simulink model "lab5_2_simulink"  (R2018a)
settings: Solver=VariableStepAuto  StartTime=0.0  StopTime=10.0  RelTol=1e-3
values from neighbouring files (symbols this model uses):
  a = 1    [lab5_2.m]
  b = 1    [lab5_1.m]    (also in lab5_2.m)
  c = -2    [lab5_2.m]
  k = 1    [lab5_2.m]
settings Model: Creator=john  LastModifiedBy=john

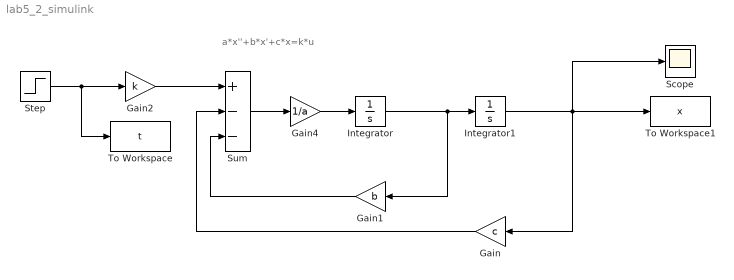
== system lab5_2_simulink ==
  note: a*x''+b*x'+c*x=k*u
  Gain : Gain  Gain=c
  Gain1 : Gain  Gain=b
  Gain2 : Gain  Gain=k
  Gain4 : Gain  Gain=1/a
  Integrator : Integrator
  Integrator1 : Integrator
  Scope : Scope
  Step : Step  After=u  SampleTime=0
  Sum : Sum  Inputs=+--
  To Workspace : ToWorkspace  VariableName=t  SaveFormat=Timeseries  SampleTime=-1
      settings: Save2DSignal=2-D array (concatenate along first dimension)
  To Workspace1 : ToWorkspace  VariableName=x  SampleTime=-1
  wires:
  Gain2/1 -> Sum/1
  Step/1 -> To Workspace/1, Gain2/1
  Sum/1 -> Gain4/1
  Gain4/1 -> Integrator/1
  Integrator/1 -> Gain1/1, Integrator1/1
  Integrator1/1 -> To Workspace1/1, Scope/1, Gain/1
  Gain1/1 -> Sum/3
  Gain/1 -> Sum/2
